simulink model "GFLIB_ControllerPIp_BAM_F16"  (Simulink 7.3)
settings: Solver=ode45  StartTime=0.0  StopTime=10.0  RelTol=1e-3
undefined symbols (not defined in the file): f16IntegGain, f16PropGain, s16IntegGainShift, s16PropGainShift
settings Model: Creator=RE004C  LastModifiedBy=RE004C
settings HardwareCC: ProdIntDivRoundTo=Zero  ProdEndianess=BigEndian  ProdHWDeviceType=Freescale->32-bit PowerPC

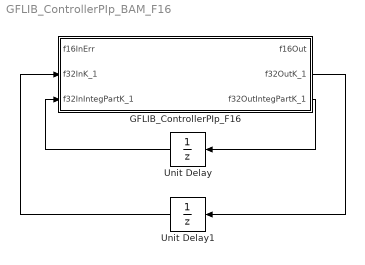
== system GFLIB_ControllerPIp_BAM_F16 ==
  GFLIB_ControllerPIp_F16 : Subsystem  mask(GFLIB_ControllerPIp_F16){f16PropGain=f16PropGain, s16PropGainShift=s16PropGainShift, f16IntegGain=f16IntegGain, s16IntegGainShift=s16IntegGainShift}
      mask help: Bit accurate model of parallel form PI controller. All parameters as well as input and output are 16-bit integers except for u16NShift parameter which is 16-bit unsigned integer.
      mask init:
      | pos = get_param(gcb, 'Position');width = pos(3) - pos(1); height = pos(4) - pos(2);tX=width/2;tY=height*0.9;
      mask Display:
      | color('black');
      | port_label('input',1,'f16InErr');
      | port_label('input',2,'f32InK_1');
      | port_label('input',3,'f32InIntegPartK_1');
      | port_label('output',1,'f16Out');
      | port_label('output',2,'f32OutK_1');
      | port_label('output',3,'f32OutIntegPartK_1');
      | color('black');
      | disp('GFLIB_ControllerPIp_F16');
      | color('blue');
      | text(tX,tY, 'BAM', 'horizontalAlignment', 'center');
  Unit Delay : UnitDelay  SampleTime=-1
  Unit Delay1 : UnitDelay  SampleTime=-1
  wires:
  GFLIB_ControllerPIp_F16/3(f32OutIntegPartK_1) -> Unit Delay/1
  Unit Delay/1 -> GFLIB_ControllerPIp_F16/3(f32InIntegPartK_1)
  GFLIB_ControllerPIp_F16/2(f32OutK_1) -> Unit Delay1/1
  Unit Delay1/1 -> GFLIB_ControllerPIp_F16/2(f32InK_1)

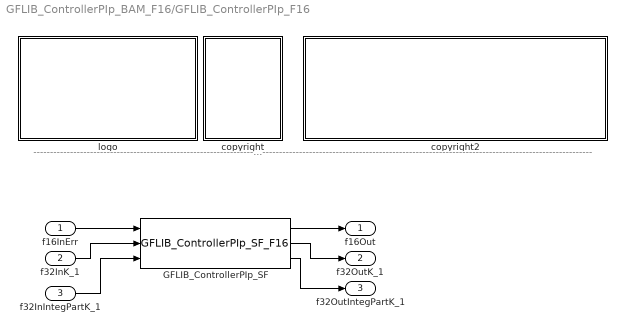
== system GFLIB_ControllerPIp_BAM_F16/GFLIB_ControllerPIp_F16 ==
  note: ---------------------------------------------------------------------------------------------------------------------------------------------------------------------------------------------------
  f16InErr : Inport  OutDataType=fixdt(1, 16)  OutScaling=2^0
  f32InK_1 : Inport  Port=2  OutDataType=fixdt(1, 16)  OutScaling=2^0
  f32InIntegPartK_1 : Inport  Port=3  OutDataType=fixdt(1, 16)  OutScaling=2^0
  GFLIB_ControllerPIp_SF : S-Function  FunctionName=GFLIB_ControllerPIp_SF_F16  Parameters=f16PropGain,s16PropGainShift,f16IntegGain,s16IntegGainShift  EnableBusSupport=off
  copyright : Subsystem
      mask Display: text(10,90,'FILE:');text(10,75,'DESRIPTION:')text(10,60,'COPYRIGHT:')text(10,45,'VERSION:')text(10,30,'DATE:')
  copyright2 : Subsystem
      mask Display: text(10,90,'GFLIB_ControllerPIp_BAM_F16.mdl');text(10,75,'Parallel form of a standard PI controller without implemented anti-windup.');text(10,60,'Freescale')text(10,45,'0.1');text(10,30,'20-Jan-2012');
  logo : Subsystem
      mask Display: image(imread('logo.jpg'))
  f16Out : Outport  OutDataType=fixdt(1, 16)  OutScaling=2^0
  f32OutK_1 : Outport  Port=2  OutDataType=fixdt(1, 16)  OutScaling=2^0
  f32OutIntegPartK_1 : Outport  Port=3  OutDataType=fixdt(1, 16)  OutScaling=2^0
  wires:
  f16InErr/1 -> GFLIB_ControllerPIp_SF/1
  GFLIB_ControllerPIp_SF/1 -> f16Out/1
  GFLIB_ControllerPIp_SF/2 -> f32OutK_1/1
  GFLIB_ControllerPIp_SF/3 -> f32OutIntegPartK_1/1
  f32InIntegPartK_1/1 -> GFLIB_ControllerPIp_SF/3
  f32InK_1/1 -> GFLIB_ControllerPIp_SF/2

== system GFLIB_ControllerPIp_BAM_F16/GFLIB_ControllerPIp_F16/copyright ==

== system GFLIB_ControllerPIp_BAM_F16/GFLIB_ControllerPIp_F16/copyright2 ==

== system GFLIB_ControllerPIp_BAM_F16/GFLIB_ControllerPIp_F16/logo ==
